simulink model "stub_model"  (R2022a)
settings: Solver=FixedStepAuto  StartTime=0.0  StopTime=600  FixedStep=0.001  RelTol=1e-3
values from neighbouring files (symbols this model uses):
  basealt = 0    [mission.m]
  basehdg = 0    [mission.m]
  baselat = 32.80045    [mission.m]
  baselon = -117.14736    [mission.m]
  uam = zeros(7, size(distsFT,2))    [mission.m]
undefined symbols (not defined in the file or in its folder): Earth, WGS84
libraries: aerolibtransform2 x4, aerolib6dof2 x1, sharedtransform x1
settings Model: Creator=cma  LastModifiedBy=cma
settings DebuggingCC: UnconnectedInputMsg=warning  UnconnectedOutputMsg=warning  UnconnectedLineMsg=warning
settings RTWCC: DLArmComputeVersion=19.05

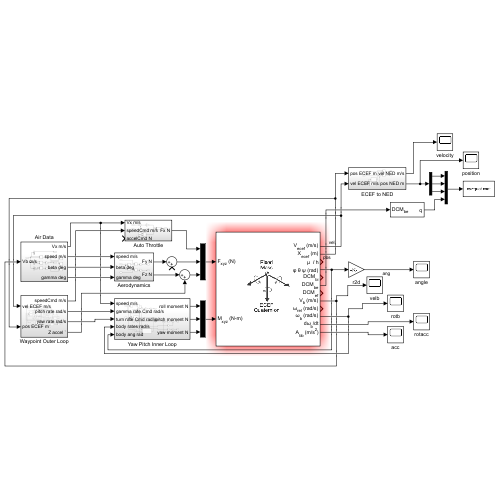
[thumbnail: Simulink's stored preview of the top-level diagram]
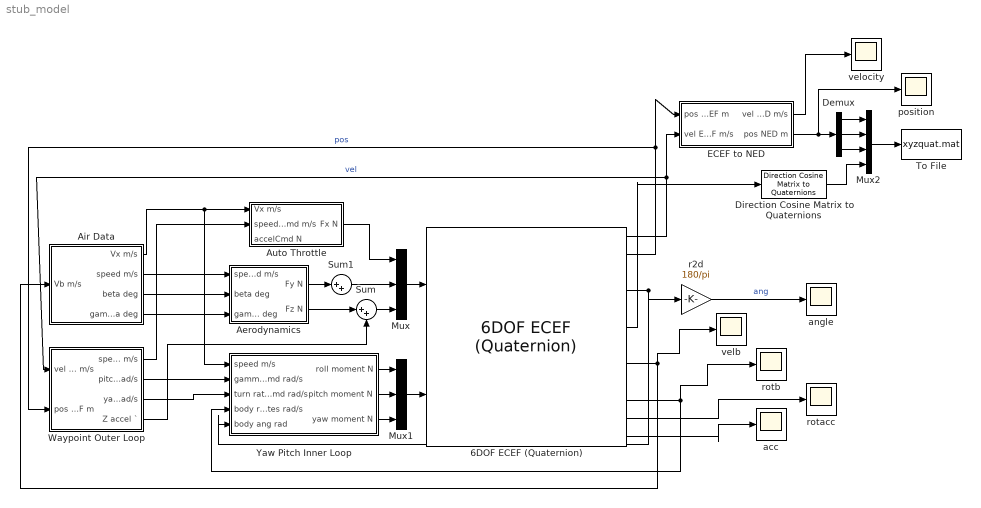
== system stub_model ==
  6DOF ECEF (Quaternion) : aerolib6dof2/6DOF ECEF (Quaternion)  units=Metric (MKS)  mtype=Fixed  xg_0=[baselat baselon basealt]  Vm_0=[0 0 0]  eul_0=[0 0 basehdg]  pm_0=[0 0 0]  mass_0=1.0  mass_e=0.5  mass_f=2.0  inertia=eye(3)  inertia_e=eye(3)  inertia_f=2*eye(3)  vre_flag=on  abi_flag=off  ptype=Earth (WGS84)  R=6378137  F=1/298.257223563  w_E=7292115e-11  angle_in=Internal  LG0=0  quat_statename=''  pm_statename=''  Vm_statename=''  posECEF_statename=''  posECI_statename=''  LG_statename=''  mass_statename=''
      settings: SourceProductBaseCode=AE
  Aerodynamics : Subsystem
  Air Data : Subsystem
  Auto Throttle : Subsystem
  Demux : Demux  Outputs=3
  Direction Cosine Matrix to Quaternions : sharedtransform/Direction Cosine Matrix  to Quaternions  aMode=0  action=None  tolerance=eps(2)
      settings: SourceProductBaseCode=AE,PW,DR,MT,VE
  ECEF to NED : Subsystem
  Mux : Mux  Inputs=3
  Mux1 : Mux  Inputs=3
  Mux2 : Mux
  Sum : Sum  Inputs=|++
  Sum1 : Sum  Inputs=|++
  To File : ToFile  Filename=xyzquat.mat  MatrixName=traj  SaveFormat=Timeseries  SampleTime=0.1
  Waypoint Outer Loop : Subsystem
  Yaw Pitch Inner Loop : Subsystem
  acc : Scope
  angle : Scope
  position : Scope
  r2d : Gain  Gain=180/pi
  rotacc : Scope
  rotb : Scope
  velb : Scope
  velocity : Scope
  wires:
  6DOF ECEF (Quaternion)/1 -> Waypoint Outer Loop/1(vel ECEF m/s), ECEF to NED/2(vel ECEF m/s)  "vel"
  6DOF ECEF (Quaternion)/2 -> ECEF to NED/1(pos ECEF m), Waypoint Outer Loop/2(pos ECEF m)  "pos"
  6DOF ECEF (Quaternion)/4 -> Yaw Pitch Inner Loop/5(body ang rad), r2d/1
  r2d/1 -> angle/1  "ang"
  6DOF ECEF (Quaternion)/12 -> acc/1
  6DOF ECEF (Quaternion)/8 -> velb/1, Air Data/1(Vb m/s)
  6DOF ECEF (Quaternion)/10 -> rotb/1, Yaw Pitch Inner Loop/4(body rates rad/s)
  6DOF ECEF (Quaternion)/11 -> rotacc/1
  Air Data/3(beta deg) -> Aerodynamics/2(beta deg)
  Air Data/4(gamma deg) -> Aerodynamics/3(gamma deg)
  Yaw Pitch Inner Loop/3(yaw moment N) -> Mux1/3
  Yaw Pitch Inner Loop/2(pitch moment N) -> Mux1/2
  Demux/3 -> Mux2/3
  Demux/1 -> Mux2/1
  Demux/2 -> Mux2/2
  6DOF ECEF (Quaternion)/6 -> Direction Cosine Matrix to Quaternions/1
  Mux2/1 -> To File/1
  Direction Cosine Matrix to Quaternions/1 -> Mux2/4
  Aerodynamics/2(Fz N) -> Sum/1
  Sum/1 -> Mux/3
  Yaw Pitch Inner Loop/1(roll moment N) -> Mux1/1
  Auto Throttle/1(Fx N) -> Mux/1
  Air Data/2(speed m/s) -> Aerodynamics/1(speed m/s)
  Air Data/1(Vx m/s) -> Yaw Pitch Inner Loop/1(speed m/s), Auto Throttle/1(Vx m/s)
  Waypoint Outer Loop/1(speedCmd m/s) -> Auto Throttle/2(speedCmd m/s)
  Waypoint Outer Loop/2(pitch rate rad/s) -> Yaw Pitch Inner Loop/2(gamma rate Cmd rad/s)
  Waypoint Outer Loop/3(yaw rate rad/s) -> Yaw Pitch Inner Loop/3(turn rate Cmd rad/s)
  Waypoint Outer Loop/4(Z accel `) -> Sum/2
  Mux/1 -> 6DOF ECEF (Quaternion)/1
  Mux1/1 -> 6DOF ECEF (Quaternion)/2
  ECEF to NED/2(pos NED m) -> position/1, Demux/1
  ECEF to NED/1(vel NED m/s) -> velocity/1
  Sum1/1 -> Mux/2
  Aerodynamics/1(Fy N) -> Sum1/1

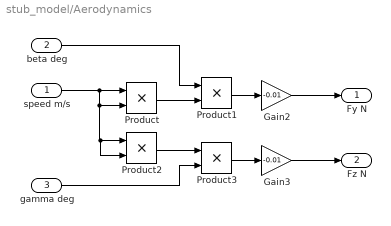
== system stub_model/Aerodynamics ==
  speed m/s : Inport
  beta deg : Inport  Port=2
  gamma deg : Inport  Port=3
  Gain2 : Gain  Gain=-0.01
  Gain3 : Gain  Gain=-0.01
  Product{,1..3} (4 alike) : Product
  Fy N : Outport
  Fz N : Outport  Port=2
  wires:
  Product2/1 -> Product3/1
  speed m/s/1 -> Product2/2, Product2/1, Product/2, Product/1
  Product/1 -> Product1/2
  Gain3/1 -> Fz N/1
  Product3/1 -> Gain3/1
  Product1/1 -> Gain2/1
  gamma deg/1 -> Product3/2
  beta deg/1 -> Product1/1
  Gain2/1 -> Fy N/1

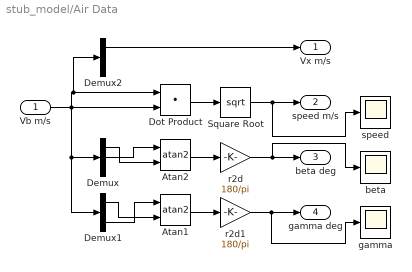
== system stub_model/Air Data ==
  Vb m/s : Inport
  Atan1 : Trigonometry  Operator=atan2
  Atan2 : Trigonometry  Operator=atan2
  Demux : Demux  Outputs=3
  Demux1 : Demux  Outputs=3
  Demux2 : Demux  Outputs=3
  Dot Product : DotProduct  OutDataTypeStr=Inherit: Inherit via internal rule
  Square Root : Sqrt
  beta : Scope
  gamma : Scope
  r2d : Gain  Gain=180/pi
  r2d1 : Gain  Gain=180/pi
  speed : Scope
  Vx m/s : Outport
  speed m/s : Outport  Port=2
  beta deg : Outport  Port=3
  gamma deg : Outport  Port=4
  wires:
  Demux1/1 -> Atan1/2
  Vb m/s/1 -> Demux2/1, Dot Product/1, Demux1/1, Demux/1, Dot Product/2
  Demux1/3 -> Atan1/1
  Atan1/1 -> r2d1/1
  r2d1/1 -> gamma/1, gamma deg/1
  Square Root/1 -> speed/1, speed m/s/1
  Demux/2 -> Atan2/1
  r2d/1 -> beta deg/1, beta/1
  Atan2/1 -> r2d/1
  Demux/1 -> Atan2/2
  Dot Product/1 -> Square Root/1
  Demux2/1 -> Vx m/s/1

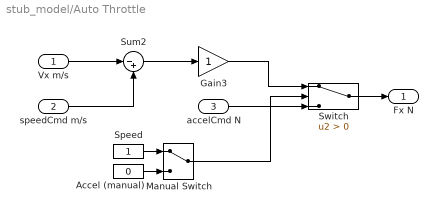
== system stub_model/Auto Throttle ==
  Vx m/s : Inport
  speedCmd m/s : Inport  Port=2
  accelCmd N : Inport  Port=3
  Accel (manual) : Constant  Value=0
  Gain3 : Gain
  Manual Switch : ManualSwitch
  Speed : Constant
  Sum2 : Sum  Inputs=|-+
  Switch : Switch  Criteria=u2 > Threshold  SaturateOnIntegerOverflow=off  InputSameDT=off
  Fx N : Outport
  wires:
  Sum2/1 -> Gain3/1
  Vx m/s/1 -> Sum2/1
  speedCmd m/s/1 -> Sum2/2
  Speed/1 -> Manual Switch/1
  Accel (manual)/1 -> Manual Switch/2
  Manual Switch/1 -> Switch/2
  Gain3/1 -> Switch/1
  Switch/1 -> Fx N/1
  accelCmd N/1 -> Switch/3

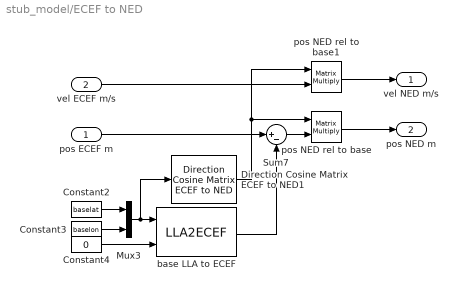
== system stub_model/ECEF to NED ==
  pos ECEF m : Inport
  vel ECEF m/s : Inport  Port=2
  Constant2 : Constant  Value=baselat
  Constant3 : Constant  Value=baselon
  Constant4 : Constant  Value=0
  Direction Cosine Matrix ECEF to NED1 : aerolibtransform2/Direction Cosine Matrix ECEF to NED
      settings: SourceProductBaseCode=AE
  Mux3 : Mux  Inputs=2
  Sum7 : Sum  Inputs=|+-
  base LLA to ECEF : LLA2ECEF
  pos NED rel to base : Product  Multiplication=Matrix(*)
  pos NED rel to base1 : Product  Multiplication=Matrix(*)
  vel NED m/s : Outport
  pos NED m : Outport  Port=2
  wires:
  Constant4/1 -> base LLA to ECEF/2
  Constant3/1 -> Mux3/2
  Constant2/1 -> Mux3/1
  Sum7/1 -> pos NED rel to base/2
  Mux3/1 -> Direction Cosine Matrix ECEF to NED1/1, base LLA to ECEF/1
  base LLA to ECEF/1 -> Sum7/2
  Direction Cosine Matrix ECEF to NED1/1 -> pos NED rel to base1/1, pos NED rel to base/1
  pos ECEF m/1 -> Sum7/1
  pos NED rel to base/1 -> pos NED m/1
  vel ECEF m/s/1 -> pos NED rel to base1/2
  pos NED rel to base1/1 -> vel NED m/s/1

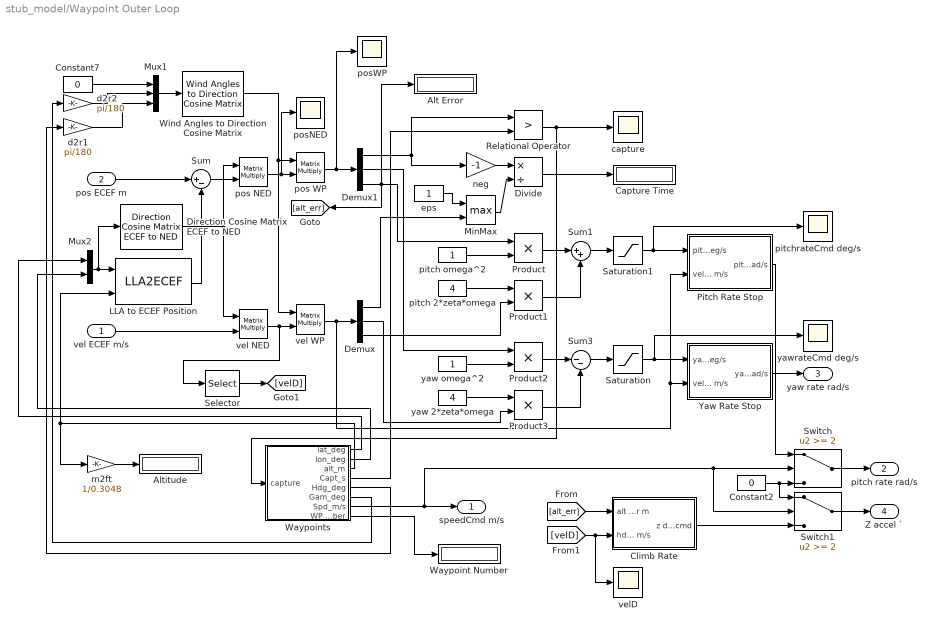
== system stub_model/Waypoint Outer Loop ==
  vel ECEF m/s : Inport
  pos ECEF m : Inport  Port=2
  Alt Error : Display
  Altitude : Display
  Capture Time : Display
  Climb Rate : Subsystem
  Constant2 : Constant  Value=0
  Constant7 : Constant  Value=0
  Demux : Demux  Outputs=3
  Demux1 : Demux  Outputs=3
  Direction Cosine Matrix ECEF to NED : aerolibtransform2/Direction Cosine Matrix ECEF to NED
      settings: SourceProductBaseCode=AE
  Divide : Product  Inputs=*/
  LLA to ECEF Position : LLA2ECEF
  MinMax : MinMax  Function=max  Inputs=2
  Mux1 : Mux  Inputs=3
  Mux2 : Mux  Inputs=2
  Pitch Rate Stop : Subsystem
  Product{,1..3} (4 alike) : Product
  Relational Operator : RelationalOperator  Operator=>  OutDataTypeStr=boolean  RndMeth=Simplest  InputSameDT=off
  Saturation : Saturate  UpperLimit=20  LowerLimit=-20
  Saturation1 : Saturate  UpperLimit=10  LowerLimit=-10
  Selector : Selector  InputPortWidth=3  IndexOptions=Index vector (dialog)  Indices=[3]  OutputSizes=1
  Sum : Sum  Inputs=|+-
  Sum1 : Sum  Inputs=|++
  Sum3 : Sum  Inputs=|--
  Switch : Switch  Threshold=2  SaturateOnIntegerOverflow=off  InputSameDT=off
  Switch1 : Switch  Threshold=2  SaturateOnIntegerOverflow=off  InputSameDT=off
  Waypoint Number : Display
  Waypoints : Subsystem
  Wind Angles to Direction Cosine Matrix : aerolibtransform2/Wind Angles to  Direction Cosine Matrix
      settings: SourceProductBaseCode=AE
  Yaw Rate Stop : Subsystem
  capture : Scope
  d2r1 : Gain  Gain=pi/180
  d2r2 : Gain  Gain=pi/180
  eps : Constant
  m2ft : Gain  Gain=1/0.3048
  neg : Gain  Gain=-1
  pitch 2*zeta*omega : Constant  Value=4
  pitch omega^2 : Constant
  pitchrateCmd deg/s : Scope
  pos NED : Product  Multiplication=Matrix(*)
  pos WP : Product  Multiplication=Matrix(*)
  posNED : Scope
  posWP : Scope
  vel NED : Product  Multiplication=Matrix(*)
  vel WP : Product  Multiplication=Matrix(*)
  velD : Scope
  yaw 2*zeta*omega : Constant  Value=4
  yaw omega^2 : Constant
  yawrateCmd deg/s : Scope
  speedCmd m/s : Outport
  pitch rate rad/s : Outport  Port=2
  yaw rate rad/s : Outport  Port=3
  Z accel ` : Outport  Port=4
  wires:
  Mux1/1 -> Wind Angles to Direction Cosine Matrix/1
  Constant7/1 -> Mux1/1
  Wind Angles to Direction Cosine Matrix/1 -> vel WP/1, pos WP/1
  pos WP/1 -> posWP/1, Demux1/1
  vel ECEF m/s/1 -> vel NED/2
  pos ECEF m/1 -> Sum/1
  Demux1/1 -> neg/1, Relational Operator/1
  Relational Operator/1 -> capture/1, Waypoints/1(capture)
  Sum1/1 -> Saturation1/1
  Product/1 -> Sum1/1
  Product1/1 -> Sum1/2
  pitch omega^2/1 -> Product/2
  pitch 2*zeta*omega/1 -> Product1/1
  Demux1/3 -> [alt_err], Alt Error/1, Product/1
  yaw 2*zeta*omega/1 -> Product3/1
  yaw omega^2/1 -> Product2/2
  Product3/1 -> Sum3/2
  Product2/1 -> Sum3/1
  Sum3/1 -> Saturation/1
  Demux1/2 -> Product2/1
  neg/1 -> Divide/1
  Divide/1 -> Capture Time/1
  Demux/3 -> Product1/2
  Demux/2 -> Product3/2
  MinMax/1 -> Divide/2
  eps/1 -> MinMax/1
  Demux/1 -> MinMax/2
  Saturation/1 -> Yaw Rate Stop/1(yaw rate Cmd deg/s), yawrateCmd deg/s/1
  vel WP/1 -> Pitch Rate Stop/2(vel WP m/s), Yaw Rate Stop/2(vel WP m/s), Demux/1
  Yaw Rate Stop/1(yaw rate rad/s) -> yaw rate rad/s/1
  Saturation1/1 -> pitchrateCmd deg/s/1, Pitch Rate Stop/1(pitch rate Cmd deg/s)
  Waypoints/1(lat_deg) -> Mux2/1
  Waypoints/5(Hdg_deg) -> d2r1/1
  Waypoints/3(alt_m) -> LLA to ECEF Position/2, m2ft/1
  Waypoints/2(lon_deg) -> Mux2/2
  Waypoints/7(Spd_m/s) -> Switch1/2, Switch/2, speedCmd m/s/1
  Waypoints/6(Gam_deg) -> d2r2/1
  d2r1/1 -> Mux1/3
  d2r2/1 -> Mux1/2
  Pitch Rate Stop/1(pitch rate rad/s) -> Switch/1
  Switch/1 -> pitch rate rad/s/1
  Constant2/1 -> Switch1/1, Switch/3
  Selector/1 -> [velD]
  [alt_err] -> Climb Rate/1(alt error m)
  [velD] -> velD/1, Climb Rate/2(hdot m/s)
  Switch1/1 -> Z accel `/1
  Climb Rate/1(z dot cmd) -> Switch1/3
  Mux2/1 -> LLA to ECEF Position/1, Direction Cosine Matrix ECEF to NED/1
  LLA to ECEF Position/1 -> Sum/2
  Sum/1 -> pos NED/2
  pos NED/1 -> posNED/1, pos WP/2
  Direction Cosine Matrix ECEF to NED/1 -> vel NED/1, pos NED/1
  vel NED/1 -> Selector/1, vel WP/2
  Waypoints/8(WP number) -> Waypoint Number/1
  m2ft/1 -> Altitude/1
  Waypoints/4(Capt_s) -> Relational Operator/2

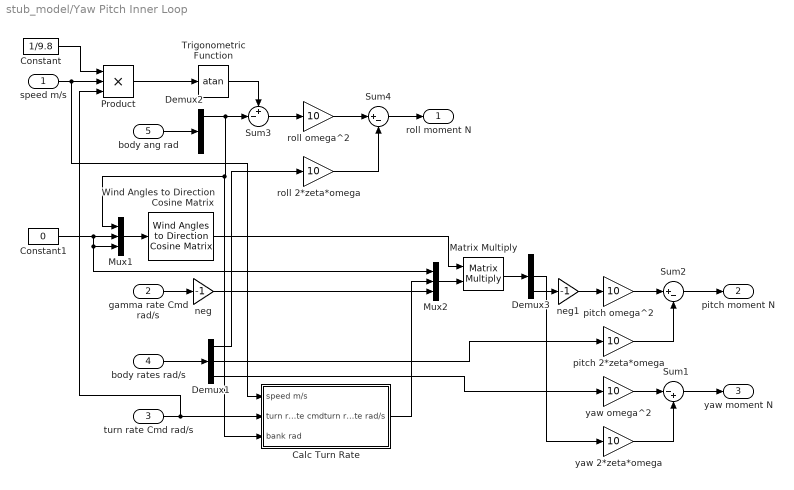
== system stub_model/Yaw Pitch Inner Loop ==
  speed m/s : Inport
  gamma rate Cmd rad/s : Inport  Port=2
  turn rate Cmd rad/s : Inport  Port=3
  body rates rad/s : Inport  Port=4
  body ang rad : Inport  Port=5
  Calc Turn Rate : Subsystem
  Constant : Constant  Value=1/9.8
  Constant1 : Constant  Value=0
  Demux1 : Demux  Outputs=3
  Demux2 : Demux  Outputs=3
  Demux3 : Demux  Outputs=3
  Matrix Multiply : Product  Multiplication=Matrix(*)
  Mux1 : Mux  Inputs=3
  Mux2 : Mux  Inputs=3
  Product : Product  Inputs=3
  Sum1 : Sum  Inputs=|-+
  Sum2 : Sum  Inputs=|+-
  Sum3 : Sum  Inputs=+-|
  Sum4 : Sum  Inputs=|+-
  Trigonometric Function : Trigonometry  Operator=atan
  Wind Angles to Direction Cosine Matrix : aerolibtransform2/Wind Angles to  Direction Cosine Matrix
      settings: SourceProductBaseCode=AE
  neg : Gain  Gain=-1
  neg1 : Gain  Gain=-1
  pitch 2*zeta*omega : Gain  Gain=10
  pitch omega^2 : Gain  Gain=10
  roll 2*zeta*omega : Gain  Gain=10
  roll omega^2 : Gain  Gain=10
  yaw 2*zeta*omega : Gain  Gain=10
  yaw omega^2 : Gain  Gain=10
  roll moment N : Outport
  pitch moment N : Outport  Port=2
  yaw moment N : Outport  Port=3
  wires:
  Sum1/1 -> yaw moment N/1
  turn rate Cmd rad/s/1 -> Calc Turn Rate/2(turn rate cmd), Product/3
  body rates rad/s/1 -> Demux1/1
  Sum2/1 -> pitch moment N/1
  body ang rad/1 -> Demux2/1
  Sum3/1 -> roll omega^2/1
  Demux2/1 -> Sum3/2, Calc Turn Rate/3(bank rad), Mux1/1
  Demux1/1 -> roll 2*zeta*omega/1
  roll omega^2/1 -> Sum4/1
  roll 2*zeta*omega/1 -> Sum4/2
  Sum4/1 -> roll moment N/1
  Trigonometric Function/1 -> Sum3/1
  Mux1/1 -> Wind Angles to Direction Cosine Matrix/1
  Wind Angles to Direction Cosine Matrix/1 -> Matrix Multiply/1
  Constant1/1 -> Mux2/1, Mux1/3, Mux1/2
  gamma rate Cmd rad/s/1 -> neg/1
  Mux2/1 -> Matrix Multiply/2
  Matrix Multiply/1 -> Demux3/1
  Demux3/2 -> yaw 2*zeta*omega/1
  Demux3/3 -> neg1/1
  neg/1 -> Mux2/3
  neg1/1 -> pitch omega^2/1
  pitch omega^2/1 -> Sum2/1
  pitch 2*zeta*omega/1 -> Sum2/2
  yaw omega^2/1 -> Sum1/1
  yaw 2*zeta*omega/1 -> Sum1/2
  Demux1/2 -> pitch 2*zeta*omega/1
  Demux1/3 -> yaw omega^2/1
  speed m/s/1 -> Calc Turn Rate/1(speed m/s), Product/2
  Constant/1 -> Product/1
  Product/1 -> Trigonometric Function/1
  Calc Turn Rate/1(turn rate rad/s) -> Mux2/2

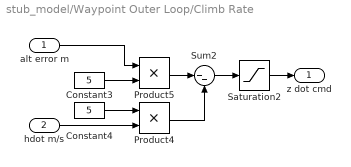
== system stub_model/Waypoint Outer Loop/Climb Rate ==
  alt error m : Inport
  hdot m/s : Inport  Port=2
  Constant3 : Constant  Value=5
  Constant4 : Constant  Value=5
  Product4 : Product
  Product5 : Product
  Saturation2 : Saturate  UpperLimit=50  LowerLimit=-50
  Sum2 : Sum  Inputs=|--
  z dot cmd : Outport
  wires:
  Constant3/1 -> Product5/2
  Product4/1 -> Sum2/2
  Product5/1 -> Sum2/1
  Sum2/1 -> Saturation2/1
  Constant4/1 -> Product4/1
  hdot m/s/1 -> Product4/2
  alt error m/1 -> Product5/1
  Saturation2/1 -> z dot cmd/1

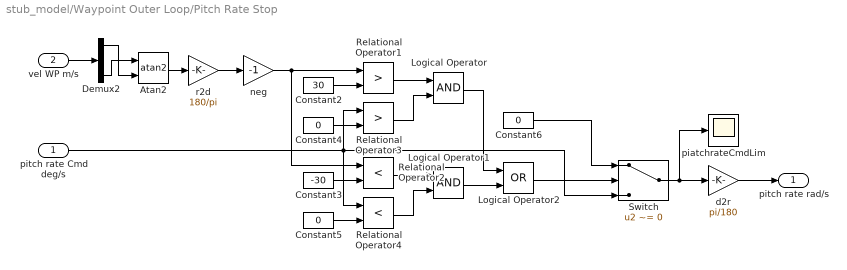
== system stub_model/Waypoint Outer Loop/Pitch Rate Stop ==
  pitch rate Cmd deg/s : Inport
  vel WP m/s : Inport  Port=2
  Atan2 : Trigonometry  Operator=atan2
  Constant2 : Constant  Value=30
  Constant3 : Constant  Value=-30
  Constant4 : Constant  Value=0
  Constant5 : Constant  Value=0
  Constant6 : Constant  Value=0
  Demux2 : Demux  Outputs=3
  Logical Operator : Logic  AllPortsSameDT=off  OutDataTypeStr=boolean
  Logical Operator1 : Logic  AllPortsSameDT=off  OutDataTypeStr=boolean
  Logical Operator2 : Logic  Operator=OR  AllPortsSameDT=off  OutDataTypeStr=boolean
  Relational Operator1 : RelationalOperator  Operator=>  OutDataTypeStr=boolean  RndMeth=Simplest  InputSameDT=off
  Relational Operator2 : RelationalOperator  Operator=<  OutDataTypeStr=boolean  RndMeth=Simplest  InputSameDT=off
  Relational Operator3 : RelationalOperator  Operator=>  OutDataTypeStr=boolean  RndMeth=Simplest  InputSameDT=off
  Relational Operator4 : RelationalOperator  Operator=<  OutDataTypeStr=boolean  RndMeth=Simplest  InputSameDT=off
  Switch : Switch  Criteria=u2 ~= 0  SaturateOnIntegerOverflow=off  InputSameDT=off
  d2r : Gain  Gain=pi/180
  neg : Gain  Gain=-1
  piatchrateCmdLim : Scope
  r2d : Gain  Gain=180/pi
  pitch rate rad/s : Outport
  wires:
  vel WP m/s/1 -> Demux2/1
  Demux2/1 -> Atan2/2
  Atan2/1 -> r2d/1
  d2r/1 -> pitch rate rad/s/1
  Constant4/1 -> Relational Operator3/2
  Logical Operator/1 -> Logical Operator2/1
  Constant2/1 -> Relational Operator1/2
  neg/1 -> Relational Operator1/1, Relational Operator2/1
  Relational Operator3/1 -> Logical Operator/2
  Relational Operator1/1 -> Logical Operator/1
  Logical Operator2/1 -> Switch/2
  Relational Operator2/1 -> Logical Operator1/1
  Constant3/1 -> Relational Operator2/2
  Constant6/1 -> Switch/1
  Relational Operator4/1 -> Logical Operator1/2
  Logical Operator1/1 -> Logical Operator2/2
  Constant5/1 -> Relational Operator4/2
  Switch/1 -> piatchrateCmdLim/1, d2r/1
  Demux2/3 -> Atan2/1
  pitch rate Cmd deg/s/1 -> Relational Operator4/1, Switch/3, Relational Operator3/1
  r2d/1 -> neg/1

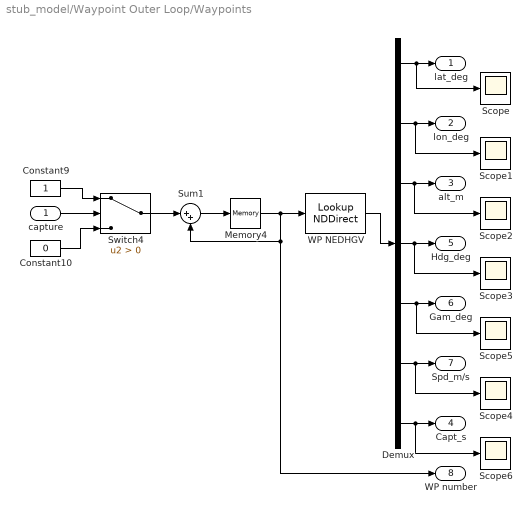
== system stub_model/Waypoint Outer Loop/Waypoints ==
  capture : Inport
  Constant10 : Constant  Value=0
  Constant9 : Constant
  Demux : Demux  Outputs=7
  Memory4 : Memory  InitialCondition=1
  Scope{,1..6} (7 alike) : Scope
  Sum1 : Sum  Inputs=|++
  Switch4 : Switch  Criteria=u2 > Threshold  SaturateOnIntegerOverflow=off  InputSameDT=off
  WP NEDHGV : LookupNDDirect  InputsSelectThisObjectFromTable=Vector  Table=uam
  lat_deg : Outport
  lon_deg : Outport  Port=2
  alt_m : Outport  Port=3
  Capt_s : Outport  Port=4
  Hdg_deg : Outport  Port=5
  Gam_deg : Outport  Port=6
  Spd_m/s : Outport  Port=7
  WP number : Outport  Port=8
  wires:
  capture/1 -> Switch4/2
  Constant9/1 -> Switch4/1
  Constant10/1 -> Switch4/3
  Switch4/1 -> Sum1/1
  Memory4/1 -> WP number/1, Sum1/2, WP NEDHGV/1
  Sum1/1 -> Memory4/1
  Demux/5 -> Scope5/1, Gam_deg/1
  Demux/4 -> Scope3/1, Hdg_deg/1
  Demux/1 -> Scope/1, lat_deg/1
  Demux/2 -> Scope1/1, lon_deg/1
  Demux/6 -> Scope4/1, Spd_m/s/1
  Demux/3 -> Scope2/1, alt_m/1
  WP NEDHGV/1 -> Demux/1
  Demux/7 -> Scope6/1, Capt_s/1

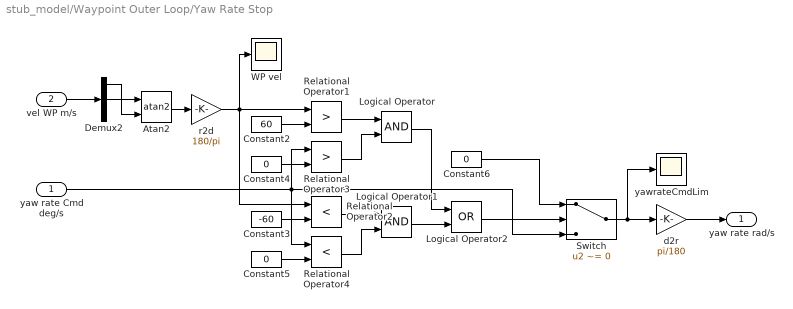
== system stub_model/Waypoint Outer Loop/Yaw Rate Stop ==
  yaw rate Cmd deg/s : Inport
  vel WP m/s : Inport  Port=2
  Atan2 : Trigonometry  Operator=atan2
  Constant2 : Constant  Value=60
  Constant3 : Constant  Value=-60
  Constant4 : Constant  Value=0
  Constant5 : Constant  Value=0
  Constant6 : Constant  Value=0
  Demux2 : Demux  Outputs=3
  Logical Operator : Logic  AllPortsSameDT=off  OutDataTypeStr=boolean
  Logical Operator1 : Logic  AllPortsSameDT=off  OutDataTypeStr=boolean
  Logical Operator2 : Logic  Operator=OR  AllPortsSameDT=off  OutDataTypeStr=boolean
  Relational Operator1 : RelationalOperator  Operator=>  OutDataTypeStr=boolean  RndMeth=Simplest  InputSameDT=off
  Relational Operator2 : RelationalOperator  Operator=<  OutDataTypeStr=boolean  RndMeth=Simplest  InputSameDT=off
  Relational Operator3 : RelationalOperator  Operator=>  OutDataTypeStr=boolean  RndMeth=Simplest  InputSameDT=off
  Relational Operator4 : RelationalOperator  Operator=<  OutDataTypeStr=boolean  RndMeth=Simplest  InputSameDT=off
  Switch : Switch  Criteria=u2 ~= 0  SaturateOnIntegerOverflow=off  InputSameDT=off
  WP vel : Scope
  d2r : Gain  Gain=pi/180
  r2d : Gain  Gain=180/pi
  yawrateCmdLim : Scope
  yaw rate rad/s : Outport
  wires:
  Switch/1 -> d2r/1, yawrateCmdLim/1
  Constant5/1 -> Relational Operator4/2
  Logical Operator1/1 -> Logical Operator2/2
  Relational Operator4/1 -> Logical Operator1/2
  yaw rate Cmd deg/s/1 -> Relational Operator3/1, Switch/3, Relational Operator4/1
  Constant6/1 -> Switch/1
  Constant3/1 -> Relational Operator2/2
  Relational Operator2/1 -> Logical Operator1/1
  Logical Operator2/1 -> Switch/2
  Relational Operator1/1 -> Logical Operator/1
  Relational Operator3/1 -> Logical Operator/2
  r2d/1 -> WP vel/1, Relational Operator2/1, Relational Operator1/1
  Constant2/1 -> Relational Operator1/2
  Logical Operator/1 -> Logical Operator2/1
  Constant4/1 -> Relational Operator3/2
  d2r/1 -> yaw rate rad/s/1
  Atan2/1 -> r2d/1
  Demux2/1 -> Atan2/2
  Demux2/2 -> Atan2/1
  vel WP m/s/1 -> Demux2/1

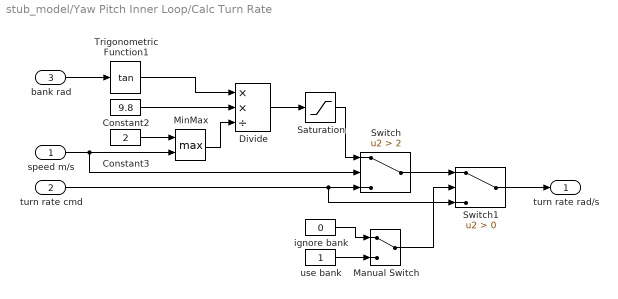
== system stub_model/Yaw Pitch Inner Loop/Calc Turn Rate ==
  speed m/s : Inport
  turn rate cmd : Inport  Port=2
  bank rad : Inport  Port=3
  Constant2 : Constant  Value=9.8
  Constant3 : Constant  Value=2
  Divide : Product  Inputs=**/
  Manual Switch : ManualSwitch
  MinMax : MinMax  Function=max  Inputs=2
  Saturation : Saturate  UpperLimit=1  LowerLimit=-1
  Switch : Switch  Criteria=u2 > Threshold  Threshold=2  SaturateOnIntegerOverflow=off  InputSameDT=off
  Switch1 : Switch  Criteria=u2 > Threshold  SaturateOnIntegerOverflow=off  InputSameDT=off
  Trigonometric Function1 : Trigonometry  Operator=tan
  ignore bank : Constant  Value=0
  use bank : Constant
  turn rate rad/s : Outport
  wires:
  bank rad/1 -> Trigonometric Function1/1
  Constant2/1 -> Divide/2
  Constant3/1 -> MinMax/1
  Trigonometric Function1/1 -> Divide/1
  MinMax/1 -> Divide/3
  Divide/1 -> Saturation/1
  speed m/s/1 -> Switch/2, MinMax/2
  Saturation/1 -> Switch/1
  turn rate cmd/1 -> Switch1/3, Switch/3
  Switch/1 -> Switch1/1
  Switch1/1 -> turn rate rad/s/1
  ignore bank/1 -> Manual Switch/1
  use bank/1 -> Manual Switch/2
  Manual Switch/1 -> Switch1/2
